simulink model "liq4MA"  (R2018b)
settings: Solver=ode45  StartTime=0.0  StopTime=100000  RelTol=1e-6  EnableMultiTasking=on
values from neighbouring files (symbols this model uses):
  A1 = d*9.9    (= 59.4)    [Lin_Analitica.m]    (also in para4nl.m)
  A2 = d*10    (= 60)    [Lin_Analitica.m]    (also in para4nl.m)
  A3 = d*10    (= 60)    [Lin_Analitica.m]    (also in para4nl.m)
  A4 = d*10    (= 60)    [Lin_Analitica.m]    (also in para4nl.m)
  k1 = 0    [Lin_Analitica.m]    (also in para4nl.m)
  k12 = 10    [para4nl.m]
  k2 = 2    [para4nl.m]
  k23 = 10    [para4nl.m]
  k3 = 0    [Lin_Analitica.m]    (also in para4nl.m)
  k34 = 10    [para4nl.m]
  k4 = 3    [para4nl.m]
  M = k3+k34*k4/sqrt(k34^2+k4^2)    [Lin_Analitica.m]    (also in ident_master.m = 1; identif.m = 5)
  PO = 12    [ident_master.m]    (also in identif.m = 15)
  qmax = 120    [para4nl.m]
  qmin = -120    [para4nl.m]
  vrh1 = 0.001*NivRuido    [para4nl.m]
  vrh2 = 0.0005*NivRuido    [para4nl.m]
  vrh3 = 0.0003*NivRuido    [para4nl.m]
  vrh4 = 0.0002*NivRuido    [para4nl.m]
  vrm = 0.001*NivRuido    [para4nl.m]
settings Model: Creator=Adolfo  LastModifiedBy=root
settings DataIOCC: LimitDataPoints=on  SaveFormat=Array  SignalLoggingSaveFormat=ModelDataLogs
settings OptimizationCC: ExpressionDepthLimit=2147483647  InitFltsAndDblsToZero=on  LifeSpan=inf
settings DebuggingCC: SaveWithParameterizedLinksMsg=none  UnderspecifiedInitializationDetection=Classic  MergeDetectMultiDrivingBlocksExec=none  SignalResolutionControl=TryResolveAllWithWarning  SolverPrmCheckMsg=warning  MultiTaskDSMMsg=warning  MultiTaskCondExecSysMsg=none  FcnCallInpInsideContextMsg=warning  StateNameClashWarn=warning  SFUnexpectedBacktrackingDiag=warning  SFNoUnconditionalDefaultTransitionDiag=warning  SFExecutionAtInitializationDiag=none
settings HardwareCC: ProdBitPerPointer=32  ProdBitPerSizeT=32  ProdBitPerPtrDiffT=32  ProdLargestAtomicFloat=None  ProdIntDivRoundTo=Undefined  ProdEndianess=Unspecified  ProdWordSize=32  ProdHWDeviceType=32-bit Generic
settings ModelReferenceCC: PropagateSignalLabelsOutOfModel=off
settings SFSimCC: SimUseLocalCustomCode=off
settings RTWCC: RTWUseLocalCustomCode=off
settings CodeAppCC: StateflowObjectComments=on
settings GRTTargetCC: TargetFcnLib=ansi_tfl_tmw.mat  TargetLangStandard=C89/C90 (ANSI)  GeneratePreprocessorConditionals=Disable all  CombineOutputUpdateFcns=off  GRTInterface=on
settings ConfigComp: CovMetricSettings=dw  CovHtmlReporting=on  CovSaveCumulativeToWorkspaceVar=on  CovSaveSingleToWorkspaceVar=on  CovExternalEMLEnable=off  CovSFcnEnable=off

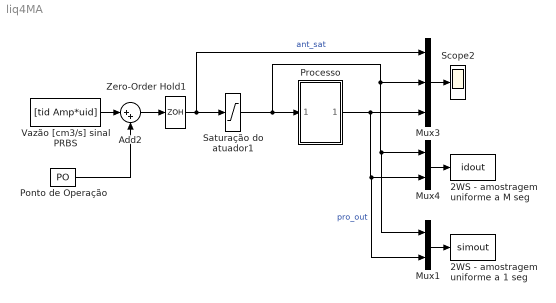
== system liq4MA ==
  2WS - amostragem uniforme a 1 seg : ToWorkspace  VariableName=simout  SaveFormat=Structure With Time  SampleTime=1
  2WS - amostragem uniforme a M seg : ToWorkspace  VariableName=idout  SaveFormat=Structure With Time  SampleTime=M
  Add2 : Sum  Inputs=|++
  Mux1 : Mux  Inputs=2
  Mux3 : Mux  Inputs=3
  Mux4 : Mux  Inputs=2
  "Ponto de Operação " : Constant  Value=PO
  Processo : Subsystem
  Saturação do atuador1 : Saturate  UpperLimit=qmax  LowerLimit=qmin
  Scope2 : Scope
  Vazão [cm3/s] sinal PRBS : FromWorkspace  VariableName=[tid Amp*uid]  SampleTime=10  Interpolate=off  OutputAfterFinalValue=Holding final value
  Zero-Order Hold1 : ZeroOrderHold  SampleTime=M
  wires:
  Mux3/1 -> Scope2/1
  Vazão [cm3/s] sinal PRBS/1 -> Add2/1
  Add2/1 -> Zero-Order Hold1/1
  "Ponto de Operação "/1 -> Add2/2
  Zero-Order Hold1/1 -> Mux3/1, Saturação do atuador1/1  "ant_sat"
  Mux4/1 -> 2WS - amostragem uniforme a M seg/1
  Saturação do atuador1/1 -> Processo/1(In1), Mux1/1, Mux4/1, Mux3/2
  Processo/1(Out1) -> Mux1/2, Mux4/2, Mux3/3  "pro_out"
  Mux1/1 -> 2WS - amostragem uniforme a 1 seg/1

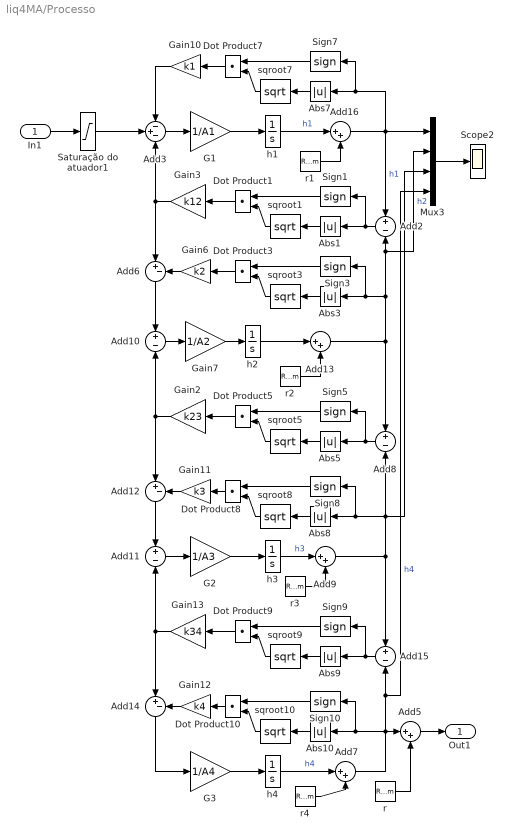
== system liq4MA/Processo ==
  In1 : Inport
  Abs{1,3,5,7..10} (7 alike) : Abs
  Add{2,8,10..11,15} (5 alike) : Sum  Inputs=+-
  Add12 : Sum  Inputs=|+-
  Add{5,7,9,13,16} (5 alike) : Sum  Inputs=|++
  Add14 : Sum  Inputs=|+-
  Add3 : Sum  Inputs=-+-
  Add6 : Sum  Inputs=|+-
  Dot Product{1,3,5,7..10} (7 alike) : DotProduct  InputSameDT=on  OutDataTypeStr=Inherit: Inherit via internal rule
  G1 : Gain  Gain=1/A1
  G2 : Gain  Gain=1/A3
  G3 : Gain  Gain=1/A4
  Gain10 : Gain  Gain=k1
  Gain11 : Gain  Gain=k3
  Gain12 : Gain  Gain=k4
  Gain13 : Gain  Gain=k34
  Gain2 : Gain  Gain=k23
  Gain3 : Gain  Gain=k12
  Gain6 : Gain  Gain=k2
  Gain7 : Gain  Gain=1/A2
  Mux3 : Mux
  Saturação do atuador1 : Saturate  UpperLimit=qmax  LowerLimit=qmin
  Scope2 : Scope
  Sign{1,3,5,7..10} (7 alike) : Signum
  h{1..4} (4 alike) : Integrator  LimitOutput=on  UpperSaturationLimit=50  LowerSaturationLimit=0
  r : RandomNumber  Variance=vrm  SampleTime=0
  r1 : RandomNumber  Variance=vrh1  Seed=400  SampleTime=0
  r2 : RandomNumber  Variance=vrh2  Seed=300  SampleTime=0
  r3 : RandomNumber  Variance=vrh3  Seed=200  SampleTime=0
  r4 : RandomNumber  Variance=vrh4  Seed=100  SampleTime=0
  sqroot{1,3,5,7..10} (7 alike) : Math  Operator=sqrt  SaturateOnIntegerOverflow=on
  Out1 : Outport
  wires:
  Add2/1 -> Abs1/1, Sign1/1
  Abs1/1 -> sqroot1/1
  Sign1/1 -> Dot Product1/1
  sqroot1/1 -> Dot Product1/2
  Dot Product1/1 -> Gain3/1
  Add3/1 -> G1/1
  Gain3/1 -> Add6/1, Add3/3
  G1/1 -> h1/1
  Abs3/1 -> sqroot3/1
  Sign3/1 -> Dot Product3/1
  sqroot3/1 -> Dot Product3/2
  Dot Product3/1 -> Gain6/1
  Gain7/1 -> h2/1
  Gain6/1 -> Add6/2
  Add8/1 -> Abs5/1, Sign5/1
  Abs5/1 -> sqroot5/1
  Sign5/1 -> Dot Product5/1
  sqroot5/1 -> Dot Product5/2
  Dot Product5/1 -> Gain2/1
  Gain2/1 -> Add10/2, Add12/1
  Abs7/1 -> sqroot7/1
  Sign7/1 -> Dot Product7/1
  sqroot7/1 -> Dot Product7/2
  Dot Product7/1 -> Gain10/1
  Gain10/1 -> Add3/1
  Add6/1 -> Add10/1
  Add10/1 -> Gain7/1
  Add11/1 -> G2/1
  G2/1 -> h3/1
  Abs8/1 -> sqroot8/1
  Sign8/1 -> Dot Product8/1
  sqroot8/1 -> Dot Product8/2
  Dot Product8/1 -> Gain11/1
  Gain11/1 -> Add12/2
  Add12/1 -> Add11/1
  Add15/1 -> Abs9/1, Sign9/1
  Abs9/1 -> sqroot9/1
  Sign9/1 -> Dot Product9/1
  sqroot9/1 -> Dot Product9/2
  Dot Product9/1 -> Gain13/1
  Gain13/1 -> Add14/1, Add11/2
  Add14/1 -> G3/1
  G3/1 -> h4/1
  Abs10/1 -> sqroot10/1
  Sign10/1 -> Dot Product10/1
  sqroot10/1 -> Dot Product10/2
  Dot Product10/1 -> Gain12/1
  Gain12/1 -> Add14/2
  r/1 -> Add5/2
  Add7/1 -> Abs10/1, Sign10/1, Mux3/4, Add15/2, Add5/1  "h4"
  h4/1 -> Add7/1  "h4"
  r4/1 -> Add7/2
  Add9/1 -> Mux3/3, Abs8/1, Sign8/1, Add8/2, Add15/1
  h3/1 -> Add9/1  "h3"
  r3/1 -> Add9/2
  Add13/1 -> Add8/1, Mux3/2, Add2/2, Abs3/1, Sign3/1  "h2"
  h2/1 -> Add13/1
  r2/1 -> Add13/2
  Add16/1 -> Mux3/1, Add2/1, Abs7/1, Sign7/1  "h1"
  h1/1 -> Add16/1  "h1"
  r1/1 -> Add16/2
  In1/1 -> Saturação do atuador1/1
  Add5/1 -> Out1/1
  Saturação do atuador1/1 -> Add3/2
  Mux3/1 -> Scope2/1
